simulink model "Projet_PSC"  (R2020b)
settings: Solver=VariableStepAuto  StartTime=0.0  StopTime=0.13  RelTol=1e-3
PreLoadFcn:
  | N = 63;
  | Ntot = N+1;
  | Np = 0.25*Ntot;
  | DIP = 4;
  | TsOFDM=0.0013;
  | Prefix = 2;
InitFcn:
  | N = 63;
  | Ntot = N+1;
  | Np = 0.25*Ntot;
  | DIP = 4;
  | TsOFDM=0.0013;
  | Prefix = 2;
undefined symbols (not defined in the file): j
libraries: dspindex x8, dspsigops x3, commutil2 x1, dspxfrm3 x1, commdigbbndpm3 x1
settings Model: Creator=nacha  LastModifiedBy=nacha

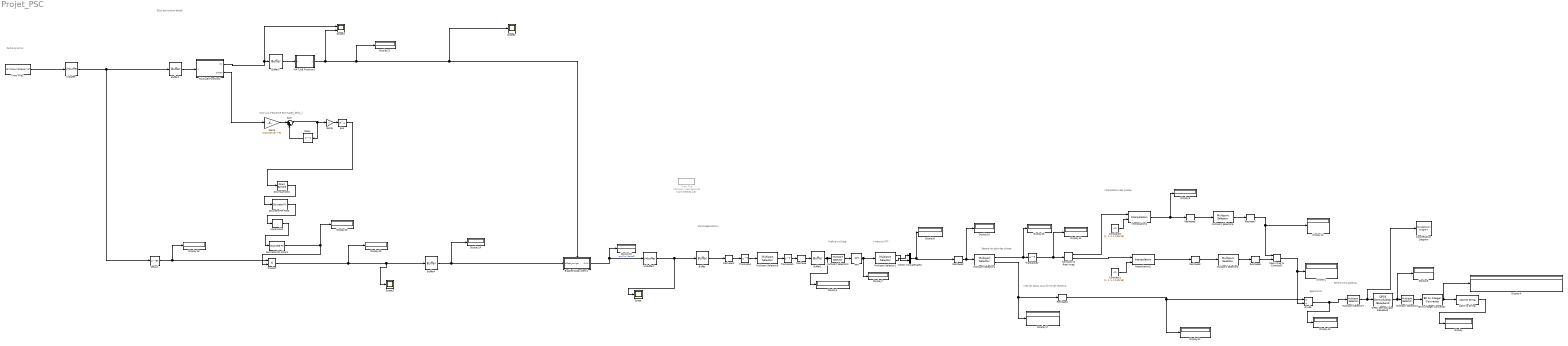
== system Projet_PSC ==
  note: Partie Egalisation :
  note: met les datas sous forme de vecteurs
  note: Préfixe cyclique:
  note: Egalisation
  note: interpolation des pilotes
  note: Inversion FFT :
  note: Sépare les data des pilotes
  note: Enlève zero padding :
  note: Bloc estimation deltaF
  note: NCO à la fréquence estimated_delta_f
  note: Partie Synchro :
  ASCII to String : ASCIIToString
  Bit to Integer Converter : commutil2/Bit to Integer Converter  nbits=8  bitOrder=MSB first  signedOutputValues=Unsigned  outDtype=uint8  outDtypeSigned=Inherit via internal rule
  Buffer : Buffer  N=(Ntot+Prefix)*10  OutputFrames=off
  Buffer1 : Buffer  N=Ntot+Prefix  OutputFrames=off
  Buffer2 : Buffer  N=660  V=659  OutputFrames=off
  Buffer3 : Buffer  N=660  V=659  OutputFrames=off
  Buffer4 : Buffer  N=660  V=659  OutputFrames=off
  Complex to Real-Imag : ComplexToRealImag
  Constant1 : Constant  Value=[1, 1, 1, 1:0.25:16]
  Constant3 : Constant  Value=[1, 1, 1, 1:0.25:16]
  Constellation Diagram : ConstellationDiagram
  Delay : Delay  DelayLength=1
  Delay1 : Delay  DelayLength=67  SampleTime=20*10^(-6)
  Discrete FIR Filter : DiscreteFir  Coefficients=(1/50)*ones(1,50)
  Discrete FIR Filter1 : DiscreteFir  Coefficients=ones(1,660)
  Display{,1..2,4..5,7..17,19,21,23..25} (21 alike) : Display
  Divide : Product  Inputs=*/
  Downsample1 : DownSample  N=660  RateOptions=Allow multirate processing
  Enabled Subsystem1 : Subsystem  TreatAsAtomicUnit=on
  Exp : Math  SaturateOnIntegerOverflow=on
  FFT : dspxfrm3/FFT  FFTImplementation=Auto  CompMethod=Table lookup  TableOpt=NEW  TableOptActive=Speed  BitRevOrder=off  Normalize=on  InheritFFTLength=on  FFTLength=64  WrapInput=on  roundingMode=Floor  overflowMode=off  firstCoeffDataTypeStr=Inherit: Same word length as input  firstCoeffLastDataTypeStr=Inherit: Same word length as input  outputMin=[]  outputMax=[]
  From File : FromFile  Commented=on  FileName=samples_message.mat  SampleTime=20e-6  ExtrapolationAfterLastDataPoint=Ground value
  From File1 : FromFile  FileName=samples_message.mat  SampleTime=50*10^(-9)  ExtrapolationAfterLastDataPoint=Ground value
  Gain4 : Gain  Gain=2*pi*20*10^(-6)
  Gain5 : Gain  Gain=-j
  Interpolation1 : dspsigops/Interpolation  InterpSource=Input port  InterpPoints=[1.1 4.8 2.67 1.6 3.2]'  InterpMode=Linear  InterpL=3  InterpR=3  InterpAlpha=0.5  InvalidMode=Clip
      settings: SourceProductBaseCode=DS
  Interpolation2 : dspsigops/Interpolation  InterpSource=Input port  InterpPoints=[1.1 4.8 2.67 1.6 3.2]'  InterpMode=Linear  InterpL=3  InterpR=3  InterpAlpha=0.5  InvalidMode=Clip
      settings: SourceProductBaseCode=DS
  MATLAB Function1 : MATLAB Function  TreatAsAtomicUnit=on
  MATLAB Function2 : MATLAB Function  TreatAsAtomicUnit=on
  Multiport Selector1 : dspindex/Multiport Selector  rowsOrCols=Rows  idxCellArray={1:Ntot/2, (Ntot/2+1):Ntot}  idxErrMode=Clip Index
  Multiport Selector2 : dspindex/Multiport Selector  rowsOrCols=Rows  idxCellArray={1:1:88}  idxErrMode=Clip Index
  Multiport Selector3 : dspindex/Multiport Selector  rowsOrCols=Rows  idxCellArray={(Prefix+1):(Ntot+Prefix)}  idxErrMode=Clip Index
  Multiport Selector4 : dspindex/Multiport Selector  rowsOrCols=Rows  idxCellArray={ DIP, 1:1:DIP-1}  idxErrMode=Clip Index
  Multiport Selector5 : dspindex/Multiport Selector  rowsOrCols=Rows  idxCellArray={ 1:1:DIP-1}  idxErrMode=Clip Index
  Multiport Selector6 : dspindex/Multiport Selector  rowsOrCols=Rows  idxCellArray={ 1:1:DIP-1}  idxErrMode=Clip Index
  Multiport Selector7 : dspindex/Multiport Selector  rowsOrCols=Rows  idxCellArray={2:N-Np+1}  idxErrMode=Clip Index
  Multiport Selector8 : dspindex/Multiport Selector  rowsOrCols=Rows  idxCellArray={ 2:1:Ntot+2}  idxErrMode=Clip Index
  Product : Product
  QPSK Demodulator Baseband : commdigbbndpm3/QPSK Demodulator Baseband  OutType=Bit  DecType=Hard decision  VarSource=Dialog  Variance=1  Dec=Gray  Ph=pi/4  outDtype1=Inherit via internal rule  outDtype2=Inherit via internal rule  derotateFactorWordLen=16  derotateFactorDataTypeStr=Inherit: Same word length as input  derotateFactorLastDataTypeStr=Inherit: Same word length as input
  Real-Imag to Complex1 : RealImagToComplex
  Reshape : Reshape
  Reshape1 : Reshape  OutputDimensionality=Customize  OutputDimensions=[Ntot+2, 10]
  Reshape2 : Reshape  OutputDimensionality=Customize  OutputDimensions=[DIP,Np]
  Reshape3 : Reshape  OutputDimensionality=Customize  OutputDimensions=[DIP, Np]
  Reshape4 : Reshape  OutputDimensions=[32, 3]
  Reshape5 : Reshape  OutputDimensions=[32, 3]
  Reshape6 : Reshape  OutputDimensionality=Customize  OutputDimensions=[DIP, Np]
  Reshape7 : Reshape  OutputDimensions=[32, 3]
  Scope : Scope
  Scope1 : Scope  NumInputPorts=2
  Scope2 : Scope
  Scope3 : Scope
  Sum : Sum  Inputs=|++
  Transpose : Math  Operator=transpose  SaturateOnIntegerOverflow=on
  Transpose1 : Math  Operator=transpose  SaturateOnIntegerOverflow=on
  Transpose2 : Math  Operator=transpose  SaturateOnIntegerOverflow=on
  Unbuffer : Unbuffer
  Unbuffer1 : Unbuffer
  Upsample1 : dspsigops/Upsample  N=660  phase=0  RateOptions=Allow multirate processing  ic=0  mode=Unused parameter value
  Vector Concatenate1 : Concatenate
  wires:
  ASCII to String/1 -> Display/1
  Transpose/1 -> Multiport Selector8/1
  Reshape1/1 -> Transpose/1
  Transpose1/1 -> Reshape/1
  Transpose2/1 -> Display11/1, Complex to Real-Imag/1
  Multiport Selector8/1 -> Transpose1/1
  Buffer1/1 -> Display1/1, Multiport Selector3/1
  Bit to Integer Converter/1 -> ASCII to String/1, Display4/1
  Multiport Selector4/2 -> Display17/1, Reshape4/1
  Constant1/1 -> Interpolation2/2
  Reshape5/1 -> Real-Imag to Complex1/2
  Multiport Selector5/1 -> Reshape5/1
  QPSK Demodulator Baseband/1 -> Display5/1, Multiport Selector2/1
  Buffer/1 -> Reshape1/1
  Complex to Real-Imag/2 -> Interpolation2/1
  Constant3/1 -> Interpolation1/2
  Multiport Selector4/1 -> Display16/1, Transpose2/1
  Multiport Selector7/1 -> Constellation Diagram/1, QPSK Demodulator Baseband/1
  Real-Imag to Complex1/1 -> Divide/2, Display2/1
  Multiport Selector2/1 -> Bit to Integer Converter/1
  Reshape7/1 -> Real-Imag to Complex1/1, Display14/1
  Divide/1 -> Multiport Selector7/1, Display13/1
  Interpolation2/1 -> Reshape3/1
  Complex to Real-Imag/1 -> Interpolation1/1
  Reshape3/1 -> Multiport Selector5/1
  FFT/1 -> Multiport Selector1/1, Display7/1
  Reshape2/1 -> Multiport Selector4/1, Display10/1
  Reshape6/1 -> Multiport Selector6/1
  Reshape/1 -> Buffer1/1
  Vector Concatenate1/1 -> Reshape2/1, Display8/1
  Multiport Selector1/2 -> Vector Concatenate1/1
  Multiport Selector3/1 -> FFT/1
  Interpolation1/1 -> Display9/1, Reshape6/1
  Reshape4/1 -> Divide/1, Display12/1
  Multiport Selector6/1 -> Reshape7/1
  Multiport Selector1/1 -> Vector Concatenate1/2
  MATLAB Function2/1(M1) -> Scope1/1, Buffer3/1
  Unbuffer/1 -> Delay1/1, Buffer2/1
  Sum/1 -> Delay/1, Gain5/1
  Buffer4/1 -> Display24/1, Enabled Subsystem1/1(offset_corrigé)
  Exp/1 -> Downsample1/1
  Delay1/1 -> Display19/1, Product/1
  Product/1 -> Display23/1, Scope3/1, Buffer4/1
  MATLAB Function1/1(y) -> Display21/1, Enabled Subsystem1/Enable, Scope2/1, Scope1/2
  Downsample1/1 -> Discrete FIR Filter/1
  Discrete FIR Filter/1 -> Upsample1/1
  Delay/1 -> Sum/2
  Enabled Subsystem1/1(Out1) -> Unbuffer1/1, Display15/1  "exp(2pi*deltaF)"
  Buffer2/1 -> MATLAB Function2/1(u)
  Buffer3/1 -> MATLAB Function1/1(u)
  Gain4/1 -> Sum/1
  Gain5/1 -> Exp/1
  Upsample1/1 -> Discrete FIR Filter1/1
  Discrete FIR Filter1/1 -> Display25/1, Product/2
  MATLAB Function2/2(deltaF) -> Gain4/1
  From File1/1 -> Unbuffer/1
  Unbuffer1/1 -> Scope/1, Buffer/1

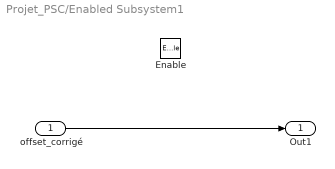
== system Projet_PSC/Enabled Subsystem1 ==
  offset_corrigé : Inport
  Enable : EnablePort  PropagateVarSize=During execution
  Out1 : Outport
  wires:
  offset_corrigé/1 -> Out1/1

== matlab function Projet_PSC/MATLAB Function2 ==
  data: u input; M1 output; deltaF output
function [M1, deltaF] = fcn(u)

T = 20*10^(-6)*660;
L = 330;
Ng = 2;
N=660;
DMAX = 660;
M = 0;
R = 0;
M1 = 0;
Mf = ones(3);
P = complex(0,0);
Rf = 0;

    for m = 1:L
        P = P + conj(u(m))*u(m+L);
    end
    M = abs(P)^2/R^2;
    for m = 1:N
        Rf = Rf+(1/2)*(abs(u(m)))^2;
    end
    
    %
    for d = 1:3
    Mf(d) = abs(P)^2/Rf^2;
    end 
    for k = -Ng:0
        M1 = M1 + (1/(1+Ng)) * Mf(k+Ng+1);
    end 
    %Mf = abs(P)^2/Rf^2;
    
   % M1 = M1 + (1/(1+Ng)) * Mf;
    
    deltaF = angle(P)/(pi*T);

== matlab function Projet_PSC/MATLAB Function1 ==
  data: u input; y output
function y = fcn(u)
max= u(1);
y=0;
for i = 4:657
    if(max<u(i))
        max=u(i);
        if 0.9<max
            if  u(i-3)<max && u(i-2)<max && u(i-1)<max && u(i+1)<=max && u(i+2)<=max && u(i+3)<=max 
                y=1;
                max = 0;
            else
                y=0;
            end

        end
    end




end
